simulink model "polydiv_test"  (R2020b)
settings: Solver=VariableStepAuto  StartTime=0.0  StopTime=inf  RelTol=1e-3
settings Model: Creator=tcbir  LastModifiedBy=tcbir

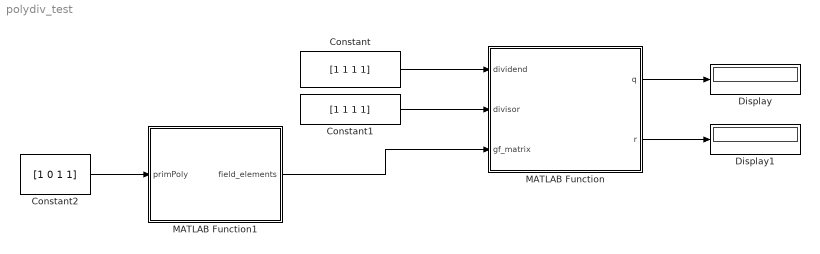
== system polydiv_test ==
  Constant : Constant  Value=[1 1 1 1]
  Constant1 : Constant  Value=[1 1 1 1]
  Constant2 : Constant  Value=[1 0 1 1]
  Display : Display
  Display1 : Display
  MATLAB Function : MATLAB Function  TreatAsAtomicUnit=on
  MATLAB Function1 : MATLAB Function  TreatAsAtomicUnit=on
  wires:
  Constant/1 -> MATLAB Function/1(dividend)
  Constant1/1 -> MATLAB Function/2(divisor)
  MATLAB Function1/1(field_elements) -> MATLAB Function/3(gf_matrix)
  Constant2/1 -> MATLAB Function1/1(primPoly)
  MATLAB Function/1(q) -> Display/1
  MATLAB Function/2(r) -> Display1/1

== matlab function polydiv_test/MATLAB Function1 ==
  data: primPoly input; field_elements output
% GenerateGF2m: generates the selected Galois Field element. The inputs should be the
% order m and the coefficients of an appropriate primitive polynomial. The generated field,
% in either binary or power notation, may be a calling parameter for each of the other
% functions. Hint: I strongly suggest that you input the coefficients in “power” notation,
% with the highest order power on the left

function field_elements  = GenerateGF2m(primPoly) %primPoly in power notation, highest order on left

m = 3;
% hard coded size of retrun matrices and gf mtrix because simulink
% whines about variable output size. Havent figured out how to fix it
% ask laberge
gf = zeros(8, 3); %there are 2^m field elements
field_elements = zeros(8, 3); %there are 2^m field elements

gfIndx = 2; %gfIndx(1) holds initial state 
numShifts = (2^m) - 1;
s_reg = zeros(1,int8(m));
s_reg(end) = 1; %rightmost element of init shr is 1
gf(1, :) = 0;%write the contents of the init shift register to the matrix of gf elements
gf(2, :) = s_reg;
for i = 2:numShifts %number of shifts corresponds to power of primitive element
    carryOut = s_reg(1);%save the value to be wrapped
    for i0 = 1:numel(s_reg)-1
        if primPoly(i0 + 1) == 1
            s_reg(i0) = xor(carryOut, s_reg(i0 + 1));
        else
            s_reg(i0) = s_reg(i0 + 1);
        end
    end
    s_reg(end) = carryOut;
    gf(i+1,:) = s_reg; %add the newly shifted register to the gf matrix
end
field_elements = gf;
end

== matlab function polydiv_test/MATLAB Function ==
  data: dividend input; q output; divisor input; gf_matrix input; r output
% Divide two polynomials over GF(2m)[x] , returning both the quotient and
% the remainder. I expect that this function will use the previous functions, as necessary.
% Hint 1: I suggest using power notation for the calling parameters and the returned
% parameter. Hint 2: this will essentially do a deconvolution with arithmetic in the Big Field.
% The MATLAB routine deconv will not do the correct algebra and so should not be used!
function [q, r] = PolyDivGF2m(dividend, divisor, gf_matrix)
m = numel(gf_matrix(1,:));
numDivs = ((numel(dividend) - 1) - (numel(divisor) - 1)); %power of dividend - power of divisor
toSubtract = -1*ones(2, numel(divisor));
quotient = -1*ones(1, numDivs);
toSubtract(1,:) = dividend(1:numel(divisor)); %initialize for first subtraction
sub_res = -1*ones(1, (numel(divisor)));
bringDwn = numel(divisor) + 1;
divs = 0; %keep track of number of iteratiions
q = zeros(numel(dividend));
%for i = 1:numDivs %is this loop redundant?
    for j = 1:(numDivs + 1) %for each element in the divisor
        in1 = toSubtract(1, 1);
        in2 = divisor(1);
        quotient = DivGF2m(in1, in2, gf_matrix);%divide the element
        for k = 1:numel(divisor)%multiply each element of dividend by quotient from prev step
            %need to do something about indexing for lower powers
            sIn1 = quotient(j);
            sIn2 = divisor(k);
            toSubtract(2, k) = MultGF2m(sIn1, sIn2, gf_matrix);
        end
        for i0 = 1:numel(divisor)%subtract
            sub_res(1,i0) = AddGF2m(toSubtract(1,i0), toSubtract(2, i0), gf_matrix);%perform the subtraction
        end
        toSubtract(1:end) = -1; %reinitialize toSubtract
        toSubtract(1, 1:numel(divisor) - 1) = sub_res(2:end); %assign the result to the next subtraction register
        if divs < numDivs %bring down number from dividend if applicable
            toSubtract(1, numel(divisor)) = dividend(bringDwn);
        end
        divs = divs + 1;
        bringDwn = bringDwn + 1;
    end
%end
r = sub_res(1,:);
%q = quotient;
q = 5;
